simulink library "mag_PD_control"  (R2016b)
settings: Solver=VariableStepAuto  StartTime=0.0  StopTime=10.0  RelTol=1e-3
undefined symbols (not defined in the file or in its folder): fsw_params
libraries: aerolibutil x2
settings Model: Creator=taylorreynolds  LastModifiedBy=taylorreynolds

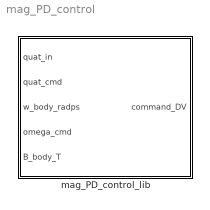
== system mag_PD_control ==
  mag_PD_control_lib : Subsystem

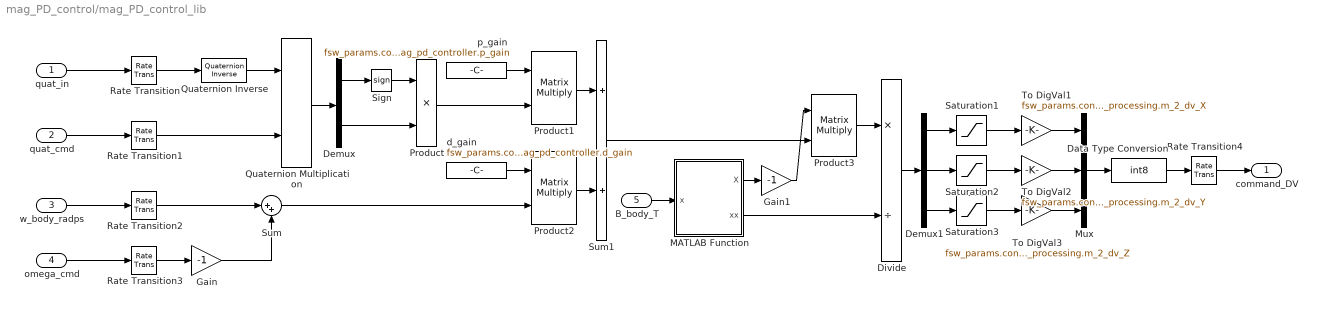
== system mag_PD_control/mag_PD_control_lib ==
  quat_in : Inport
  quat_cmd : Inport  Port=2
  w_body_radps : Inport  Port=3
  omega_cmd : Inport  Port=4
  B_body_T : Inport  Port=5
  Data Type Conversion : DataTypeConversion  OutDataTypeStr=int8
  Demux : Demux  Outputs=[1 3]
  Demux1 : Demux  Outputs=3
  Divide : Product  Inputs=*/
  Gain : Gain  Gain=-1
  Gain1 : Gain  Gain=-1
  MATLAB Function : MATLAB Function  TreatAsAtomicUnit=on
  Mux : Mux  Inputs=3
  Product : Product
  Product1 : Product  Multiplication=Matrix(*)
  Product2 : Product  Multiplication=Matrix(*)
  Product3 : Product  Multiplication=Matrix(*)
  Quaternion Inverse : aerolibutil/Quaternion Inverse
  Quaternion Multiplication : aerolibutil/Quaternion Multiplication
  Rate Transition{,1..3} (4 alike) : RateTransition  OutPortSampleTime=fsw_params.control.mag_pd_controller.sample_time_s
  Rate Transition4 : RateTransition
  Saturation1 : Saturate  UpperLimit=fsw_params.actuators.magnetorquer.max_dipole_x  LowerLimit=-fsw_params.actuators.magnetorquer.max_dipole_x
  Saturation2 : Saturate  UpperLimit=fsw_params.actuators.magnetorquer.max_dipole_y  LowerLimit=-fsw_params.actuators.magnetorquer.max_dipole_y
  Saturation3 : Saturate  UpperLimit=fsw_params.actuators.magnetorquer.max_dipole_z  LowerLimit=-fsw_params.actuators.magnetorquer.max_dipole_z
  Sign : Signum
  Sum : Sum  Inputs=|++
  Sum1 : Sum
  To DigVal1 : Gain  Gain=fsw_params.control.cmd_processing.m_2_dv_X
  To DigVal2 : Gain  Gain=fsw_params.control.cmd_processing.m_2_dv_Y
  To DigVal3 : Gain  Gain=fsw_params.control.cmd_processing.m_2_dv_Z
  d_gain : Constant  Value=fsw_params.control.mag_pd_controller.d_gain  SampleTime=fsw_params.control.mag_pd_controller.sample_time_s
  p_gain : Constant  Value=fsw_params.control.mag_pd_controller.p_gain  SampleTime=fsw_params.control.mag_pd_controller.sample_time_s
  command_DV : Outport
  wires:
  quat_in/1 -> Rate Transition/1
  w_body_radps/1 -> Rate Transition2/1
  omega_cmd/1 -> Rate Transition3/1
  quat_cmd/1 -> Rate Transition1/1
  Rate Transition4/1 -> command_DV/1
  Rate Transition/1 -> Quaternion Inverse/1
  Quaternion Inverse/1 -> Quaternion Multiplication/1
  Rate Transition1/1 -> Quaternion Multiplication/2
  Quaternion Multiplication/1 -> Demux/1
  Demux/1 -> Sign/1
  Sign/1 -> Product/1
  Demux/2 -> Product/2
  Product/1 -> Product1/2
  p_gain/1 -> Product1/1
  Rate Transition3/1 -> Gain/1
  Gain/1 -> Sum/2
  Rate Transition2/1 -> Sum/1
  d_gain/1 -> Product2/1
  Sum/1 -> Product2/2
  Product1/1 -> Sum1/1
  Product2/1 -> Sum1/2
  Sum1/1 -> Product3/2
  B_body_T/1 -> MATLAB Function/1(x)
  Product3/1 -> Divide/1
  MATLAB Function/2(xx) -> Divide/2
  Divide/1 -> Demux1/1
  Demux1/1 -> Saturation1/1
  Demux1/3 -> Saturation3/1
  Demux1/2 -> Saturation2/1
  Saturation1/1 -> To DigVal1/1
  Saturation2/1 -> To DigVal2/1
  Saturation3/1 -> To DigVal3/1
  Mux/1 -> Data Type Conversion/1
  To DigVal3/1 -> Mux/3
  To DigVal2/1 -> Mux/2
  To DigVal1/1 -> Mux/1
  Data Type Conversion/1 -> Rate Transition4/1
  MATLAB Function/1(X) -> Gain1/1
  Gain1/1 -> Product3/1

== matlab function mag_PD_control/mag_PD_control_lib/MATLAB Function ==
  data: x input; X output; xx output
function [X,xx]   = skew( x )
%--------------------------------------------------------------------------
% UW HuskySat-1, ADCS Subsystem
%
% Transforms a vector into a skew symmetric matrix and outputs its norm
% square.
%
% T. Reynolds
%--------------------------------------------------------------------------
% #codegen
% FLAG = 0;

X   = [0 -x(3) x(2);x(3) 0 -x(1);-x(2) x(1) 0];
xx  = dot(x,x);

% if( abs(xx) < 1e-8 )
%     FLAG = -1;
% end

end
